simulink model "BBcca1b"  (R2020a)
settings: Solver=VariableStepAuto  StartTime=0.0  StopTime=5  RelTol=1e-3  EnableMultiTasking=on
InitFcn:
  | k = 1e6;
  | d = 500;
  | beta = 0.002;
  | g = 9.81;
settings Model: ExtModeAutoUpdateStatusClock=off  Creator=peter  LastModifiedBy=peter
settings DataIOCC: LimitDataPoints=on  SaveFormat=Array  SignalLoggingSaveFormat=ModelDataLogs  ReturnWorkspaceOutputs=off  SignalLoggingName=sigsOut  Refine=10
settings OptimizationCC: BooleanDataType=off  ExpressionDepthLimit=2147483647  LifeSpan=inf
settings DebuggingCC: SaveWithParameterizedLinksMsg=none  UnderspecifiedInitializationDetection=Classic  MergeDetectMultiDrivingBlocksExec=none  SignalResolutionControl=TryResolveAllWithWarning  MultiTaskDSMMsg=warning  MultiTaskCondExecSysMsg=none  FcnCallInpInsideContextMsg=warning  StateNameClashWarn=warning  SFUnexpectedBacktrackingDiag=warning  SFNoUnconditionalDefaultTransitionDiag=warning  SFExecutionAtInitializationDiag=none  ArithmeticOperatorsInVariantConditions=warning
settings HardwareCC: ProdBitPerPointer=32  ProdBitPerSizeT=32  ProdBitPerPtrDiffT=32  ProdLargestAtomicFloat=None  ProdIntDivRoundTo=Undefined  ProdEndianess=Unspecified  ProdWordSize=32  ProdHWDeviceType=32-bit Generic  TargetUnknown=on
settings ModelReferenceCC: PropagateSignalLabelsOutOfModel=off
settings SFSimCC: SimUseLocalCustomCode=off  CustomCodeUndefinedFunction=UseInterfaceOnly
settings RTWCC: RTWUseLocalCustomCode=off
settings CodeAppCC: StateflowObjectComments=on
settings GRTTargetCC: TargetLangStandard=C89/C90 (ANSI)  CombineOutputUpdateFcns=off  GRTInterface=on
settings ConfigComp: CovMetricSettings=dw  CovHtmlReporting=on  CovSaveCumulativeToWorkspaceVar=on  CovSaveSingleToWorkspaceVar=on  CovExternalEMLEnable=off

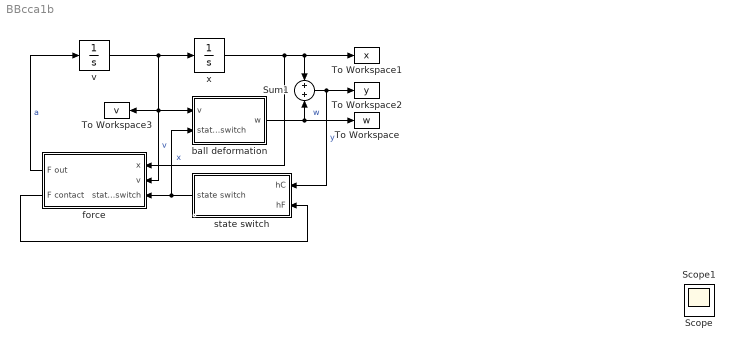
== system BBcca1b ==
  note: .
  Sum1 : Sum  Inputs=+|+
  To Workspace : ToWorkspace  VariableName=w  SaveFormat=Timeseries  SampleTime=-1
  To Workspace1 : ToWorkspace  VariableName=x  SaveFormat=Timeseries  SampleTime=-1
  To Workspace2 : ToWorkspace  VariableName=y  SaveFormat=Timeseries  SampleTime=-1
  To Workspace3 : ToWorkspace  VariableName=v  SaveFormat=Timeseries  SampleTime=-1
  ball deformation : Subsystem  mask{k=k, d=d}
      mask help:
      | This block discribes the ball deformation. It depends on the state of the system and switches between free fall and contact phases.
      | In the free fall phase the ball behaves like an elastic spring with the parameters k and d.
      | In the contact phase the deformation depends from the velocity.
  force : Subsystem  mask{beta=beta, k=k, d=d, g=g}
      mask help: This block discribes the inner forces in the system and switches between the contact force and the friction force.
  state switch : Subsystem
  v : Integrator  LowerSaturationLimit=0
  x : Integrator  InitialCondition=10  LowerSaturationLimit=0
  Scope : Scope
  Scope1 : Scope
  wires:
  v/1 -> To Workspace3/1, ball deformation/1(v), force/2(v), x/1  "v"
  x/1 -> To Workspace1/1, Sum1/1, force/1(x)  "x"
  force/1(F out) -> v/1  "a"
  state switch/1(state switch) -> ball deformation/2(state switch), force/3(state switch)
  Sum1/1 -> To Workspace2/1, state switch/1(hC)  "y"
  force/2(F contact) -> state switch/2(hF)
  ball deformation/1(w) -> To Workspace/1, Sum1/2  "w"

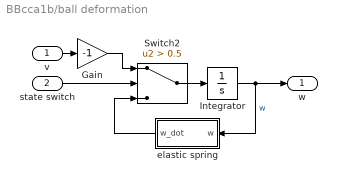
== system BBcca1b/ball deformation ==
  v : Inport
  state switch : Inport  Port=2
  Gain : Gain  Gain=-1
  Integrator : Integrator
  Switch2 : Switch  Criteria=u2 > Threshold  Threshold=0.5
  elastic spring : Subsystem  mask{k=k, d=d}
  w : Outport
  wires:
  Integrator/1 -> w/1, elastic spring/1(w)  "w"
  Switch2/1 -> Integrator/1
  Gain/1 -> Switch2/1
  v/1 -> Gain/1
  elastic spring/1(w_dot) -> Switch2/3
  state switch/1 -> Switch2/2

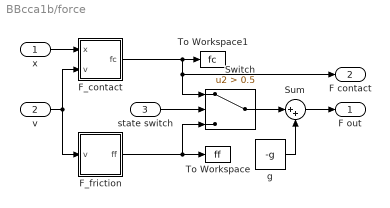
== system BBcca1b/force ==
  x : Inport
  v : Inport  Port=2
  state switch : Inport  Port=3
  F_contact : Subsystem  mask{d=d, k=k}
  F_friction : Subsystem  mask{beta=beta}
  Sum : Sum  Inputs=|++
  Switch : Switch  Criteria=u2 > Threshold  Threshold=0.5
  To Workspace : ToWorkspace  VariableName=ff  SaveFormat=Timeseries  SampleTime=-1
  To Workspace1 : ToWorkspace  VariableName=fc  SaveFormat=Timeseries  SampleTime=-1
  g : Constant  Value=-g
  F out : Outport
  F contact : Outport  Port=2
  wires:
  v/1 -> F_contact/2(v), F_friction/1(v)
  state switch/1 -> Switch/2
  F_contact/1(fc) -> Switch/1, F contact/1, To Workspace1/1
  x/1 -> F_contact/1(x)
  F_friction/1(ff) -> To Workspace/1, Switch/3
  Sum/1 -> F out/1
  Switch/1 -> Sum/1
  g/1 -> Sum/2

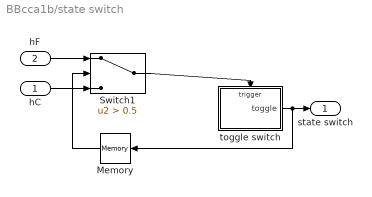
== system BBcca1b/state switch ==
  hC : Inport
  hF : Inport  Port=2
  Memory : Memory
  Switch1 : Switch  Criteria=u2 > Threshold  Threshold=0.5
  toggle switch : Subsystem
  state switch : Outport
  wires:
  Switch1/1 -> toggle switch/Trigger
  toggle switch/1(toggle) -> state switch/1, Memory/1
  hF/1 -> Switch1/1
  Memory/1 -> Switch1/2
  hC/1 -> Switch1/3

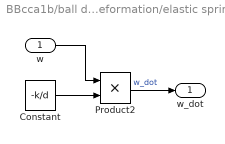
== system BBcca1b/ball deformation/elastic spring ==
  w : Inport
  Constant : Constant  Value=-k/d
  Product2 : Product
  w_dot : Outport  VectorParamsAs1DForOutWhenUnconnected=off
  wires:
  w/1 -> Product2/1
  Product2/1 -> w_dot/1  "w_dot"
  Constant/1 -> Product2/2

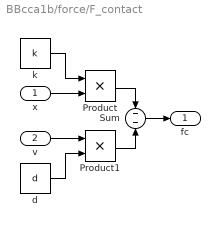
== system BBcca1b/force/F_contact ==
  x : Inport
  v : Inport  Port=2
  Product : Product
  Product1 : Product
  Sum : Sum  Inputs=--
  d : Constant  Value=d
  k : Constant  Value=k
  fc : Outport  VectorParamsAs1DForOutWhenUnconnected=off
  wires:
  k/1 -> Product/1
  d/1 -> Product1/2
  Sum/1 -> fc/1
  Product1/1 -> Sum/2
  Product/1 -> Sum/1
  v/1 -> Product1/1
  x/1 -> Product/2

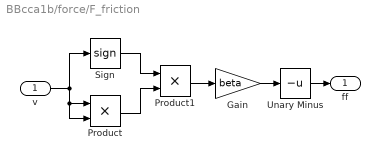
== system BBcca1b/force/F_friction ==
  v : Inport
  Gain : Gain  Gain=beta
  Product : Product
  Product1 : Product
  Sign : Signum
  Unary Minus : UnaryMinus
  ff : Outport  VectorParamsAs1DForOutWhenUnconnected=off
  wires:
  v/1 -> Sign/1, Product/2, Product/1
  Product1/1 -> Gain/1
  Sign/1 -> Product1/1
  Product/1 -> Product1/2
  Gain/1 -> Unary Minus/1
  Unary Minus/1 -> ff/1

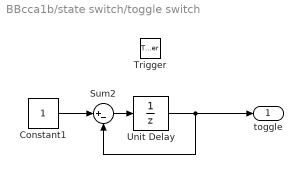
== system BBcca1b/state switch/toggle switch ==
  Trigger : TriggerPort  TriggerType=falling  VariantControl=Variant  InitialTriggerSignalState=positive  PortDimensions=1
  Constant1 : Constant
  Sum2 : Sum  Inputs=|+-
  Unit Delay : UnitDelay  SampleTime=-1  HasFrameUpgradeWarning=on
  toggle : Outport  VectorParamsAs1DForOutWhenUnconnected=off
  wires:
  Constant1/1 -> Sum2/1
  Sum2/1 -> Unit Delay/1
  Unit Delay/1 -> toggle/1, Sum2/2
